simulink model "CSE_SIMULINK_BLOCK_DIAGRAM_NO2"  (R2023a)
settings: Solver=VariableStepAuto  StartTime=0.0  StopTime=10  RelTol=1e-3
undefined symbols (not defined in the file): G1D, G1N, G2D, G2N, G3D, G3N, G4D, G4N, H1D, H1N, H2D, H2N, H3D, H3N, tden, tnum
settings Model: Creator=Ray  LastModifiedBy=Ray

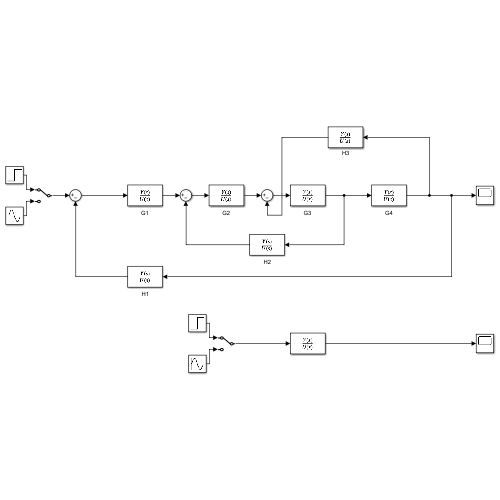
[thumbnail: Simulink's stored preview of the top-level diagram]
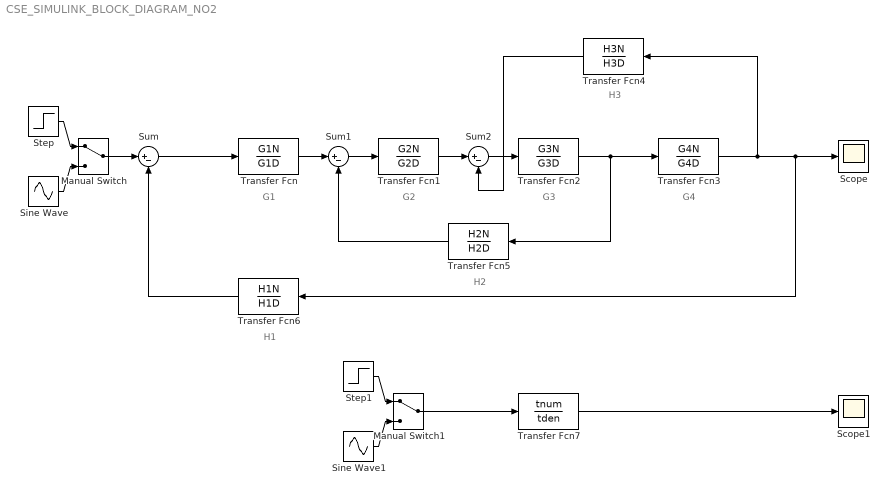
== system CSE_SIMULINK_BLOCK_DIAGRAM_NO2 ==
  note: G2
  note: G1
  note: G3
  note: G4
  note: H1
  note: H2
  note: H3
  Manual Switch : ManualSwitch
  Manual Switch1 : ManualSwitch
  Scope : Scope
  Scope1 : Scope
  Sine Wave : Sin  SampleTime=0
  Sine Wave1 : Sin  SampleTime=0
  Step : Step  SampleTime=0
  Step1 : Step  SampleTime=0
  Sum : Sum  Inputs=|+-
  Sum1 : Sum  Inputs=|+-
  Sum2 : Sum  Inputs=|+-
  Transfer Fcn : TransferFcn  Numerator=G1N  Denominator=G1D
  Transfer Fcn1 : TransferFcn  Numerator=G2N  Denominator=G2D
  Transfer Fcn2 : TransferFcn  Numerator=G3N  Denominator=G3D
  Transfer Fcn3 : TransferFcn  Numerator=G4N  Denominator=G4D
  Transfer Fcn4 : TransferFcn  Numerator=H3N  Denominator=H3D
  Transfer Fcn5 : TransferFcn  Numerator=H2N  Denominator=H2D
  Transfer Fcn6 : TransferFcn  Numerator=H1N  Denominator=H1D
  Transfer Fcn7 : TransferFcn  Numerator=tnum  Denominator=tden
  wires:
  Sum/1 -> Transfer Fcn/1
  Sum1/1 -> Transfer Fcn1/1
  Transfer Fcn/1 -> Sum1/1
  Transfer Fcn1/1 -> Sum2/1
  Sum2/1 -> Transfer Fcn2/1
  Transfer Fcn6/1 -> Sum/2
  Transfer Fcn5/1 -> Sum1/2
  Transfer Fcn4/1 -> Sum2/2
  Transfer Fcn3/1 -> Transfer Fcn4/1, Transfer Fcn6/1, Scope/1
  Transfer Fcn2/1 -> Transfer Fcn5/1, Transfer Fcn3/1
  Step/1 -> Manual Switch/1
  Sine Wave/1 -> Manual Switch/2
  Manual Switch/1 -> Sum/1
  Sine Wave1/1 -> Manual Switch1/2
  Step1/1 -> Manual Switch1/1
  Manual Switch1/1 -> Transfer Fcn7/1
  Transfer Fcn7/1 -> Scope1/1
